simulink model "simscape_quadcopter_readtime_LQR_V1_2020a"  (R2022b)
settings: Solver=ode8  StartTime=0.0  StopTime=200  FixedStep=0.002  RelTol=1e-3
values from neighbouring files (symbols this model uses):
  C = [ 1  0  0  0  0  0 ... (first row only)    [LQR_QUADCOPTER_6STATE.m]    (also in LQR_QUADCOPTER_8STATE.m = [ 1     0     0     0     0     0     0     0)
  g = 9.81    [LQR_QUADCOPTER_6STATE.m]
  K_LQR_GOC = lqr(A,B,Q,R)    [LQR_QUADCOPTER_6STATE.m]
  m = 1.7    [LQR_QUADCOPTER_6STATE.m]
  pitch_init = 0    [LQR_QUADCOPTER_6STATE.m]    (also in LQR_QUADCOPTER_8STATE.m)
  roll_init = 0    [LQR_QUADCOPTER_6STATE.m]    (also in LQR_QUADCOPTER_8STATE.m)
  v_pitch_init = 0    [LQR_QUADCOPTER_6STATE.m]    (also in LQR_QUADCOPTER_8STATE.m)
  v_roll_init = 0    [LQR_QUADCOPTER_6STATE.m]    (also in LQR_QUADCOPTER_8STATE.m)
  v_x_init = 0    [LQR_QUADCOPTER_6STATE.m]    (also in LQR_QUADCOPTER_8STATE.m)
  v_y_init = 0    [LQR_QUADCOPTER_6STATE.m]    (also in LQR_QUADCOPTER_8STATE.m)
  v_yaw_init = 0    [LQR_QUADCOPTER_6STATE.m]    (also in LQR_QUADCOPTER_8STATE.m)
  v_z_init = 0    [LQR_QUADCOPTER_6STATE.m]    (also in LQR_QUADCOPTER_8STATE.m)
  x_init = 0    [LQR_QUADCOPTER_6STATE.m]    (also in LQR_QUADCOPTER_8STATE.m)
  y_init = 0    [LQR_QUADCOPTER_6STATE.m]    (also in LQR_QUADCOPTER_8STATE.m)
  yaw_init = 0    [LQR_QUADCOPTER_6STATE.m]    (also in LQR_QUADCOPTER_8STATE.m)
  z_init = 0    [LQR_QUADCOPTER_6STATE.m]    (also in LQR_QUADCOPTER_8STATE.m)
undefined symbols (not defined in the file or in its folder): drone_leg, X, Y, Z
libraries: sm_lib x55, nesl_utility x12, simulink x1
(part 1 of 2)
settings Model: Creator=tridu  LastModifiedBy=tridu
settings SolverCC: AlgebraicLoopSolver=TrustRegion
settings OptimizationCC: GainParamInheritBuiltInType=on

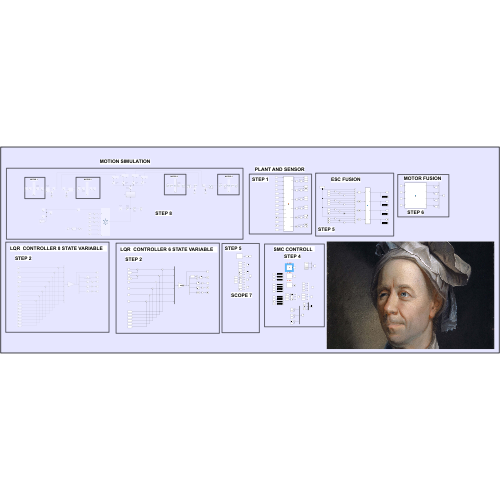
[thumbnail: Simulink's stored preview of the top-level diagram]
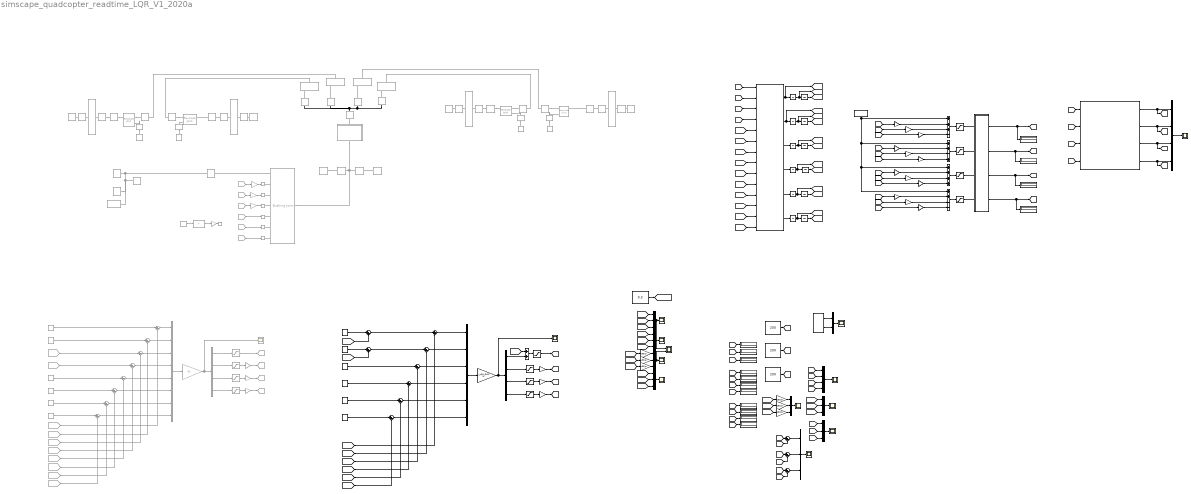
== system simscape_quadcopter_readtime_LQR_V1_2020a ==
  note: Z SP
  note: ARM 2
  note: ARM 2
  note: MOTOR 2
  note: MOTOR 3
  note: ARM 2
  note: MOTOR 1
  note: ARM 2
  note: ARM 2
  note: STEP 1
  note: STEP 5
  note: STEP 5
  note: MOTOR 4
  note: ARM 2
  note: SCOPE 7
  note: ARM 2
  note: ESC FUSION
  note: ARM 2
  note: STEP 8
  note: STEP 6
  note: PLANT AND SENSOR
  note: MOTION SIMULATION
  note: STEP 2
  note: LQR CONTROLLER 8 STATE VARIABLE
  note: ARM 2
  note: ARM 2
  note: MOTOR FUSION
  note: ARM 2
  note: STEP 2
  note: LQR CONTROLLER 6 STATE VARIABLE
  note: ARM 2
  note: SMC CONTROLL
  note: STEP 4
  note: X SP
  note: Y SP
  " Arm1" : sm_lib/Body Elements/File Solid  Commented=on  ExtGeomFileName=C:\Users\tridu\OneDrive\Máy tính\Code Matlad\quadcopter\CAD\Geometry\quadcopter_drone_arm.stp  UnitType=FromFile  ExtGeomFileUnits=m  StepReaderType=HEX  ExportConvexHullGeometry=off  InertiaType=Custom  Mass=0.0589152  MassUnits=kg  CenterOfMass=[-4.85019e-05, -0.00435236, -0.00536926]  CenterOfMassUnits=m  MomentsOfInertia=[0.000263222, 0.000260855, 1.23093e-05]  MomentsOfInertiaUnits=kg*m^2  ProductsOfInertia=[1.89459e-06, 5.49897e-08, 2.10429e-08]  ProductsOfInertiaUnits=kg*m^2  BasedOnType=Density  Density=1  DensityUnits=g/cm^3  DoExposeReferenceFrame=off  SerializedFrames=<Frames><Frame><Id>Frame1</Id><Value><Name>port</Name><Origin><Source>GeometricFeature</Source><FeatureName>planar surface 13</FeatureName></Origin><PrimaryAxis><DefinedDirection>-Z</DefinedDirection><Source>ReferenceFrame</Source><SourceDirection>+Z</SourceDirection><FeatureName></FeatureName></PrimaryAxis><SecondaryAxis><DefinedDirection>-X</DefinedDirection><Source>ReferenceFrame</Source><SourceDirection>+X</SourceDirection><FeatureName></FeatureName></SecondaryAxis></Value></Frame><Frame><Id>Frame2</Id><Value><Name>F2</Name><Origin><Source>GeometricFeature</Source><FeatureName>planar surface 4</FeatureName></Origin><PrimaryAxis><DefinedDirection>+Z</DefinedDirection><Source>ReferenceFrame</Source><SourceDirection>+Z</SourceDirection><FeatureName></FeatureName></PrimaryAxis><SecondaryAxis><DefinedDirection>+X</DefinedDirection><Source>ReferenceFrame</Source><SourceDirection>+X</SourceDirection><FeatureName></FeatureName></SecondaryAxis></Value></Frame><Frame><Id>Frame4</Id><Value><Name>Foot</Name><Origin><Source>GeometricFeature</Source><FeatureName>planar surface 62</FeatureName></Origin><PrimaryAxis><DefinedDirection>+Z</DefinedDirection><Source>ReferenceFrame</Source><SourceDirection>+Z</SourceDirection><FeatureName></FeatureName></PrimaryAxis><SecondaryAxis><DefinedDirection>+X</DefinedDirection><Source>ReferenceFrame</Source><SourceDirection>+X</SourceDirection><FeatureName></FeatureName></SecondaryAxis></Value></Frame></Frames>  GraphicType=FromGeometry  MarkerShape=Sphere  MarkerSize=10  GraphicVisPropType=SimpleVisualProperties  GraphicDiffuseColor=[1.0 0.0 0.2]  GraphicSpecularColor=[0.5 0.5 0.5 1.0]  GraphicAmbientColor=[0.15 0.15 0.15 1.0]  GraphicEmissiveColor=[0.0 0.0 0.0 1.0]  GraphicShininess=75  GraphicOpacity=1.0
  " Arm2" : sm_lib/Body Elements/File Solid  Commented=on  ExtGeomFileName=C:\Users\tridu\OneDrive\Máy tính\Code Matlad\quadcopter\CAD\Geometry\quadcopter_drone_arm.stp  UnitType=FromFile  ExtGeomFileUnits=m  StepReaderType=HEX  ExportConvexHullGeometry=off  InertiaType=Custom  Mass=0.0589152  MassUnits=kg  CenterOfMass=[-4.85019e-05, -0.00435236, -0.00536926]  CenterOfMassUnits=m  MomentsOfInertia=[0.000263222, 0.000260855, 1.23093e-05]  MomentsOfInertiaUnits=kg*m^2  ProductsOfInertia=[1.89459e-06, 5.49897e-08, 2.10429e-08]  ProductsOfInertiaUnits=kg*m^2  BasedOnType=Density  Density=1  DensityUnits=g/cm^3  DoExposeReferenceFrame=off  SerializedFrames=<Frames><Frame><Id>Frame1</Id><Value><Name>port</Name><Origin><Source>GeometricFeature</Source><FeatureName>planar surface 13</FeatureName></Origin><PrimaryAxis><DefinedDirection>-Z</DefinedDirection><Source>ReferenceFrame</Source><SourceDirection>+Z</SourceDirection><FeatureName></FeatureName></PrimaryAxis><SecondaryAxis><DefinedDirection>-X</DefinedDirection><Source>ReferenceFrame</Source><SourceDirection>+X</SourceDirection><FeatureName></FeatureName></SecondaryAxis></Value></Frame><Frame><Id>Frame2</Id><Value><Name>F2</Name><Origin><Source>GeometricFeature</Source><FeatureName>planar surface 4</FeatureName></Origin><PrimaryAxis><DefinedDirection>+Z</DefinedDirection><Source>ReferenceFrame</Source><SourceDirection>+Z</SourceDirection><FeatureName></FeatureName></PrimaryAxis><SecondaryAxis><DefinedDirection>+X</DefinedDirection><Source>ReferenceFrame</Source><SourceDirection>+X</SourceDirection><FeatureName></FeatureName></SecondaryAxis></Value></Frame><Frame><Id>Frame4</Id><Value><Name>Foot</Name><Origin><Source>GeometricFeature</Source><FeatureName>planar surface 62</FeatureName></Origin><PrimaryAxis><DefinedDirection>+Z</DefinedDirection><Source>ReferenceFrame</Source><SourceDirection>+Z</SourceDirection><FeatureName></FeatureName></PrimaryAxis><SecondaryAxis><DefinedDirection>+X</DefinedDirection><Source>ReferenceFrame</Source><SourceDirection>+X</SourceDirection><FeatureName></FeatureName></SecondaryAxis></Value></Frame></Frames>  GraphicType=FromGeometry  MarkerShape=Sphere  MarkerSize=10  GraphicVisPropType=SimpleVisualProperties  GraphicDiffuseColor=[1.0 0.0 0.2]  GraphicSpecularColor=[0.5 0.5 0.5 1.0]  GraphicAmbientColor=[0.15 0.15 0.15 1.0]  GraphicEmissiveColor=[0.0 0.0 0.0 1.0]  GraphicShininess=75  GraphicOpacity=1.0
  Add : Sum
  Add1 : Sum  Inputs=+++-
  Add3 : Sum  Inputs=++-+
  Add4 : Sum  Inputs=++++
  Add5 : Sum  Inputs=++--
  Arm1 : sm_lib/Body Elements/File Solid  Commented=on  ExtGeomFileName=C:\Users\tridu\OneDrive\Máy tính\Code Matlad\quadcopter\CAD\Geometry\quadcopter_drone_arm.stp  UnitType=FromFile  ExtGeomFileUnits=m  StepReaderType=HEX  ExportConvexHullGeometry=off  InertiaType=Custom  Mass=0.0589152  MassUnits=kg  CenterOfMass=[-4.85019e-05, -0.00435236, -0.00536926]  CenterOfMassUnits=m  MomentsOfInertia=[0.000263222, 0.000260855, 1.23093e-05]  MomentsOfInertiaUnits=kg*m^2  ProductsOfInertia=[1.89459e-06, 5.49897e-08, 2.10429e-08]  ProductsOfInertiaUnits=kg*m^2  BasedOnType=Density  Density=1  DensityUnits=g/cm^3  DoExposeReferenceFrame=off  SerializedFrames=<Frames><Frame><Id>Frame1</Id><Value><Name>port</Name><Origin><Source>GeometricFeature</Source><FeatureName>planar surface 13</FeatureName></Origin><PrimaryAxis><DefinedDirection>-Z</DefinedDirection><Source>ReferenceFrame</Source><SourceDirection>+Z</SourceDirection><FeatureName></FeatureName></PrimaryAxis><SecondaryAxis><DefinedDirection>-X</DefinedDirection><Source>ReferenceFrame</Source><SourceDirection>+X</SourceDirection><FeatureName></FeatureName></SecondaryAxis></Value></Frame><Frame><Id>Frame2</Id><Value><Name>F2</Name><Origin><Source>GeometricFeature</Source><FeatureName>planar surface 4</FeatureName></Origin><PrimaryAxis><DefinedDirection>+Z</DefinedDirection><Source>ReferenceFrame</Source><SourceDirection>+Z</SourceDirection><FeatureName></FeatureName></PrimaryAxis><SecondaryAxis><DefinedDirection>+X</DefinedDirection><Source>ReferenceFrame</Source><SourceDirection>+X</SourceDirection><FeatureName></FeatureName></SecondaryAxis></Value></Frame><Frame><Id>Frame3</Id><Value><Name>Foot</Name><Origin><Source>GeometricFeature</Source><FeatureName>planar surface 62</FeatureName></Origin><PrimaryAxis><DefinedDirection>+Z</DefinedDirection><Source>ReferenceFrame</Source><SourceDirection>+Z</SourceDirection><FeatureName></FeatureName></PrimaryAxis><SecondaryAxis><DefinedDirection>+X</DefinedDirection><Source>ReferenceFrame</Source><SourceDirection>+X</SourceDirection><FeatureName></FeatureName></SecondaryAxis></Value></Frame></Frames>  GraphicType=FromGeometry  MarkerShape=Sphere  MarkerSize=10  GraphicVisPropType=SimpleVisualProperties  GraphicDiffuseColor=[1.0 1.0 1.0]  GraphicSpecularColor=[0.5 0.5 0.5 1.0]  GraphicAmbientColor=[0.15 0.15 0.15 1.0]  GraphicEmissiveColor=[0.0 0.0 0.0 1.0]  GraphicShininess=75  GraphicOpacity=1.0
  Arm2 : sm_lib/Body Elements/File Solid  Commented=on  ExtGeomFileName=C:\Users\tridu\OneDrive\Máy tính\Code Matlad\quadcopter\CAD\Geometry\quadcopter_drone_arm.stp  UnitType=FromFile  ExtGeomFileUnits=m  StepReaderType=HEX  ExportConvexHullGeometry=off  InertiaType=Custom  Mass=0.0589152  MassUnits=kg  CenterOfMass=[-4.85019e-05, -0.00435236, -0.00536926]  CenterOfMassUnits=m  MomentsOfInertia=[0.000263222, 0.000260855, 1.23093e-05]  MomentsOfInertiaUnits=kg*m^2  ProductsOfInertia=[1.89459e-06, 5.49897e-08, 2.10429e-08]  ProductsOfInertiaUnits=kg*m^2  BasedOnType=Density  Density=1  DensityUnits=g/cm^3  DoExposeReferenceFrame=off  SerializedFrames=<Frames><Frame><Id>Frame1</Id><Value><Name>port</Name><Origin><Source>GeometricFeature</Source><FeatureName>planar surface 13</FeatureName></Origin><PrimaryAxis><DefinedDirection>-Z</DefinedDirection><Source>ReferenceFrame</Source><SourceDirection>+Z</SourceDirection><FeatureName></FeatureName></PrimaryAxis><SecondaryAxis><DefinedDirection>-X</DefinedDirection><Source>ReferenceFrame</Source><SourceDirection>+X</SourceDirection><FeatureName></FeatureName></SecondaryAxis></Value></Frame><Frame><Id>Frame2</Id><Value><Name>F2</Name><Origin><Source>GeometricFeature</Source><FeatureName>planar surface 4</FeatureName></Origin><PrimaryAxis><DefinedDirection>+Z</DefinedDirection><Source>ReferenceFrame</Source><SourceDirection>+Z</SourceDirection><FeatureName></FeatureName></PrimaryAxis><SecondaryAxis><DefinedDirection>+X</DefinedDirection><Source>ReferenceFrame</Source><SourceDirection>+X</SourceDirection><FeatureName></FeatureName></SecondaryAxis></Value></Frame><Frame><Id>Frame3</Id><Value><Name>Foot</Name><Origin><Source>GeometricFeature</Source><FeatureName>planar surface 62</FeatureName></Origin><PrimaryAxis><DefinedDirection>+Z</DefinedDirection><Source>ReferenceFrame</Source><SourceDirection>+Z</SourceDirection><FeatureName></FeatureName></PrimaryAxis><SecondaryAxis><DefinedDirection>+X</DefinedDirection><Source>ReferenceFrame</Source><SourceDirection>+X</SourceDirection><FeatureName></FeatureName></SecondaryAxis></Value></Frame></Frames>  GraphicType=FromGeometry  MarkerShape=Sphere  MarkerSize=10  GraphicVisPropType=SimpleVisualProperties  GraphicDiffuseColor=[1.0 1.0 1.0]  GraphicSpecularColor=[0.5 0.5 0.5 1.0]  GraphicAmbientColor=[0.15 0.15 0.15 1.0]  GraphicEmissiveColor=[0.0 0.0 0.0 1.0]  GraphicShininess=75  GraphicOpacity=1.0
  Body : Subsystem  Commented=on
  Bushing Joint : sm_lib/Joints/Bushing Joint  Commented=on  JointMode=Normal  SenseConstraintForce=off  SenseConstraintForceX=off  SenseConstraintForceY=off  SenseConstraintForceZ=off  SenseConstraintTorque=off  SenseConstraintTorqueX=off  SenseConstraintTorqueY=off  SenseConstraintTorqueZ=off  SenseTotalForce=off  SenseTotalForceX=off  SenseTotalForceY=off  SenseTotalForceZ=off  SenseTotalTorque=off  SenseTotalTorqueX=off  SenseTotalTorqueY=off  SenseTotalTorqueZ=off  CompositeWrenchDir=FollowerOnBase  CompositeWrenchFrame=BaseFrame  PxEquilibriumPosition=0  PxEquilibriumPositionUnits=m  PxSpringStiffness=0  PxSpringStiffnessUnits=N/m  PxDampingCoefficient=0  PxDampingCoefficientUnits=N/(m/s)  PxTorqueActuationMode=ComputedTorque  PxMotionActuationMode=InputMotion  PxSensePosition=off  PxSenseVelocity=off  PxSenseAcceleration=off  PxSenseTorqueForce=off  PxSenseLowerLimitTorqueForce=off  PxSenseUpperLimitTorqueForce=off  PxLowerLimitSpecify=off  PxLowerLimitBound=-1  PxLowerLimitBoundUnits=m  PxLowerLimitStiffness=1e6  PxLowerLimitStiffnessUnits=N/m  PxLowerLimitDamping=1e3  PxLowerLimitDampingUnits=N/(m/s)  PxLowerLimitTransitionRegionWidth=1e-4  PxLowerLimitTransitionRegionWidthUnits=m  PxUpperLimitSpecify=off  PxUpperLimitBound=1  PxUpperLimitBoundUnits=m  PxUpperLimitStiffness=1e6  PxUpperLimitStiffnessUnits=N/m  PxUpperLimitDamping=1e3  PxUpperLimitDampingUnits=N/(m/s)  PxUpperLimitTransitionRegionWidth=1e-4  PxUpperLimitTransitionRegionWidthUnits=m  PxPositionTargetSpecify=off  PxPositionTargetPriority=High  PxPositionTargetValue=0  PxPositionTargetValueUnits=m  PxVelocityTargetSpecify=off  PxVelocityTargetPriority=High  PxVelocityTargetValue=0  PxVelocityTargetValueUnits=m/s  PyEquilibriumPosition=0  PyEquilibriumPositionUnits=m  PySpringStiffness=0  PySpringStiffnessUnits=N/m  PyDampingCoefficient=0  PyDampingCoefficientUnits=N/(m/s)  PyTorqueActuationMode=ComputedTorque  PyMotionActuationMode=InputMotion  PySensePosition=off  PySenseVelocity=off  PySenseAcceleration=off  PySenseTorqueForce=off  PySenseLowerLimitTorqueForce=off  PySenseUpperLimitTorqueForce=off  PyLowerLimitSpecify=off  PyLowerLimitBound=-1  PyLowerLimitBoundUnits=m  PyLowerLimitStiffness=1e6  PyLowerLimitStiffnessUnits=N/m  PyLowerLimitDamping=1e3  PyLowerLimitDampingUnits=N/(m/s)  PyLowerLimitTransitionRegionWidth=1e-4  PyLowerLimitTransitionRegionWidthUnits=m  PyUpperLimitSpecify=off  PyUpperLimitBound=1  PyUpperLimitBoundUnits=m  PyUpperLimitStiffness=1e6  PyUpperLimitStiffnessUnits=N/m  PyUpperLimitDamping=1e3  PyUpperLimitDampingUnits=N/(m/s)  PyUpperLimitTransitionRegionWidth=1e-4  PyUpperLimitTransitionRegionWidthUnits=m  PyPositionTargetSpecify=off  PyPositionTargetPriority=High  PyPositionTargetValue=0  PyPositionTargetValueUnits=m  PyVelocityTargetSpecify=off  PyVelocityTargetPriority=High  PyVelocityTargetValue=0  PyVelocityTargetValueUnits=m/s  PzEquilibriumPosition=0  PzEquilibriumPositionUnits=m  PzSpringStiffness=0  PzSpringStiffnessUnits=N/m  PzDampingCoefficient=0  PzDampingCoefficientUnits=N/(m/s)  PzTorqueActuationMode=ComputedTorque  PzMotionActuationMode=InputMotion  PzSensePosition=off  PzSenseVelocity=off  PzSenseAcceleration=off  PzSenseTorqueForce=off  PzSenseLowerLimitTorqueForce=off  PzSenseUpperLimitTorqueForce=off  PzLowerLimitSpecify=off  PzLowerLimitBound=-1  PzLowerLimitBoundUnits=m  PzLowerLimitStiffness=1e6  PzLowerLimitStiffnessUnits=N/m  PzLowerLimitDamping=1e3  PzLowerLimitDampingUnits=N/(m/s)  PzLowerLimitTransitionRegionWidth=1e-4  PzLowerLimitTransitionRegionWidthUnits=m  PzUpperLimitSpecify=off  PzUpperLimitBound=1  PzUpperLimitBoundUnits=m  PzUpperLimitStiffness=1e6  PzUpperLimitStiffnessUnits=N/m  PzUpperLimitDamping=1e3  PzUpperLimitDampingUnits=N/(m/s)  PzUpperLimitTransitionRegionWidth=1e-4  PzUpperLimitTransitionRegionWidthUnits=m  PzPositionTargetSpecify=off  PzPositionTargetPriority=High  PzPositionTargetValue=0  PzPositionTargetValueUnits=m  PzVelocityTargetSpecify=off  PzVelocityTargetPriority=High  PzVelocityTargetValue=0  PzVelocityTargetValueUnits=m/s  RxEquilibriumPosition=0  RxEquilibriumPositionUnits=deg  RxSpringStiffness=0  RxSpringStiffnessUnits=N*m/deg  RxDampingCoefficient=0  RxDampingCoefficientUnits=N*m/(deg/s)  RxTorqueActuationMode=ComputedTorque  RxMotionActuationMode=InputMotion  RxSensePosition=off  RxSenseVelocity=off  RxSenseAcceleration=off  RxSenseTorqueForce=off  RxSenseLowerLimitTorqueForce=off  RxSenseUpperLimitTorqueForce=off  RxLowerLimitSpecify=off  RxLowerLimitBound=-90  RxLowerLimitBoundUnits=deg  RxLowerLimitStiffness=1e4  RxLowerLimitStiffnessUnits=N*m/deg  RxLowerLimitDamping=10  RxLowerLimitDampingUnits=N*m/(deg/s)  RxLowerLimitTransitionRegionWidth=0.1  RxLowerLimitTransitionRegionWidthUnits=deg  RxUpperLimitSpecify=off  RxUpperLimitBound=90  RxUpperLimitBoundUnits=deg  RxUpperLimitStiffness=1e4  RxUpperLimitStiffnessUnits=N*m/deg  RxUpperLimitDamping=10  RxUpperLimitDampingUnits=N*m/(deg/s)  RxUpperLimitTransitionRegionWidth=0.1  RxUpperLimitTransitionRegionWidthUnits=deg  RxPositionTargetSpecify=off  RxPositionTargetPriority=High  RxPositionTargetValue=0  RxPositionTargetValueUnits=deg  RxVelocityTargetSpecify=off  RxVelocityTargetPriority=High  RxVelocityTargetValue=0  RxVelocityTargetValueUnits=deg/s  RyEquilibriumPosition=0  RyEquilibriumPositionUnits=deg  RySpringStiffness=0  RySpringStiffnessUnits=N*m/deg  RyDampingCoefficient=0  RyDampingCoefficientUnits=N*m/(deg/s)  RyTorqueActuationMode=ComputedTorque  RyMotionActuationMode=InputMotion  RySensePosition=off  RySenseVelocity=off  RySenseAcceleration=off  RySenseTorqueForce=off  RySenseLowerLimitTorqueForce=off  RySenseUpperLimitTorqueForce=off  RyLowerLimitSpecify=off  RyLowerLimitBound=-90  RyLowerLimitBoundUnits=deg  RyLowerLimitStiffness=1e4  RyLowerLimitStiffnessUnits=N*m/deg  RyLowerLimitDamping=10  RyLowerLimitDampingUnits=N*m/(deg/s)  RyLowerLimitTransitionRegionWidth=0.1  RyLowerLimitTransitionRegionWidthUnits=deg  RyUpperLimitSpecify=off  RyUpperLimitBound=90  RyUpperLimitBoundUnits=deg  RyUpperLimitStiffness=1e4  RyUpperLimitStiffnessUnits=N*m/deg  RyUpperLimitDamping=10  RyUpperLimitDampingUnits=N*m/(deg/s)  RyUpperLimitTransitionRegionWidth=0.1  RyUpperLimitTransitionRegionWidthUnits=deg  RyPositionTargetSpecify=off  RyPositionTargetPriority=High  RyPositionTargetValue=0  RyPositionTargetValueUnits=deg  RyVelocityTargetSpecify=off  RyVelocityTargetPriority=High  RyVelocityTargetValue=0  RyVelocityTargetValueUnits=deg/s  RzEquilibriumPosition=0  RzEquilibriumPositionUnits=deg  RzSpringStiffness=0  RzSpringStiffnessUnits=N*m/deg  RzDampingCoefficient=0  RzDampingCoefficientUnits=N*m/(deg/s)  RzTorqueActuationMode=ComputedTorque  RzMotionActuationMode=InputMotion  RzSensePosition=off  RzSenseVelocity=off  RzSenseAcceleration=off  RzSenseTorqueForce=off  RzSenseLowerLimitTorqueForce=off  RzSenseUpperLimitTorqueForce=off  RzLowerLimitSpecify=off  RzLowerLimitBound=-90  RzLowerLimitBoundUnits=deg  RzLowerLimitStiffness=1e4  RzLowerLimitStiffnessUnits=N*m/deg  RzLowerLimitDamping=10  RzLowerLimitDampingUnits=N*m/(deg/s)  RzLowerLimitTransitionRegionWidth=0.1  RzLowerLimitTransitionRegionWidthUnits=deg  RzUpperLimitSpecify=off  RzUpperLimitBound=90  RzUpperLimitBoundUnits=deg  RzUpperLimitStiffness=1e4  RzUpperLimitStiffnessUnits=N*m/deg  RzUpperLimitDamping=10  RzUpperLimitDampingUnits=N*m/(deg/s)  RzUpperLimitTransitionRegionWidth=0.1  RzUpperLimitTransitionRegionWidthUnits=deg  RzPositionTargetSpecify=off  RzPositionTargetPriority=High  RzPositionTargetValue=0  RzPositionTargetValueUnits=deg  RzVelocityTargetSpecify=off  RzVelocityTargetPriority=High  RzVelocityTargetValue=0  RzVelocityTargetValueUnits=deg/s
  Cap{1..4} (4 alike) : sm_lib/Body Elements/File Solid  Commented=on  ExtGeomFileName=C:\Users\tridu\OneDrive\Máy tính\Code Matlad\quadcopter\CAD\Geometry\quadcopter_drone_motor_cap.stp  UnitType=FromFile  ExtGeomFileUnits=m  StepReaderType=HEX  ExportConvexHullGeometry=off  InertiaType=Custom  Mass=0.000930841  MassUnits=kg  CenterOfMass=[0 0.00200877 0]  CenterOfMassUnits=m  MomentsOfInertia=[1.32154e-08, 2.22535e-08, 1.32154e-08]  MomentsOfInertiaUnits=kg*m^2  ProductsOfInertia=[0 0 0]  ProductsOfInertiaUnits=kg*m^2  BasedOnType=Density  Density=1  DensityUnits=g/cm^3  DoExposeReferenceFrame=on  SerializedFrames=<Frames/>  GraphicType=FromGeometry  MarkerShape=Sphere  MarkerSize=10  GraphicVisPropType=AdvancedVisualProperties  GraphicDiffuseColor=[0.05 0.05 0.05]  GraphicSpecularColor=[0.5 0.5 0.5 1.0]  GraphicAmbientColor=[0.15 0.15 0.15 1.0]  GraphicEmissiveColor=[0.0 0.0 0.0 1.0]  GraphicShininess=40  GraphicOpacity=1.0
  Constant : Constant  Value=1.7*9.81/4
  Constant1 : Constant  Commented=on  Value=-1
  Constant13 : Constant  Commented=on  Value=100
  Constant{4,14..17} (5 alike) : Constant  Commented=on  Value=0
  Constant{2..3,23,25..27} (6 alike) : Constant  Value=0
  Constant28 : Constant  Commented=on
  Constant29 : Constant  Value=200
  Constant31 : Constant  Value=200
  Constant36 : Constant  Value=200
  Constant37 : Constant  Commented=on
  Constant38 : Constant  Commented=on
  Constant7 : Constant  Commented=on  Value=-1
  Demux1 : Demux  Commented=on
  Demux2 : Demux
  Display{,1..10,14..17} (15 alike) : Display
  From18 : From  Commented=on  GotoTag=z  TagVisibility=global
  From19 : From  Commented=on  GotoTag=roll  TagVisibility=global
  From20 : From  Commented=on  GotoTag=pitch  TagVisibility=global
  From21 : From  Commented=on  GotoTag=yaw  TagVisibility=global
  From22 : From  Commented=on  GotoTag=roll  TagVisibility=global
  From23 : From  Commented=on  GotoTag=yawdot  TagVisibility=global
  From24 : From  Commented=on  GotoTag=x  TagVisibility=global
  From25 : From  Commented=on  GotoTag=y  TagVisibility=global
  From26 : From  Commented=on  GotoTag=pitchdot  TagVisibility=global
  From27 : From  Commented=on  GotoTag=rolldot  TagVisibility=global
  From28 : From  Commented=on  GotoTag=yaw  TagVisibility=global
  From29 : From  Commented=on  GotoTag=pitch  TagVisibility=global
  From57 : From  Commented=on  GotoTag=zdot  TagVisibility=global
  From60 : From  Commented=on  GotoTag=z  TagVisibility=global
  From71 : From  Commented=on  GotoTag=roll_SP  TagVisibility=global
  From72 : From  Commented=on  GotoTag=pitch_SP  TagVisibility=global
  Gain1 : Gain  Commented=on  Gain=1/110
  Gain{8..12,14,16,18} (8 alike) : Gain  Gain=1/4
  Gain{13,15,17,19} (4 alike) : Gain  Gain=1/2
  Gain2 : Gain  Commented=on  Gain=1/100
  Gain20 : Gain  Gain=0.3
  Gain21 : Gain  Commented=on  Gain=|  Multiplication=Matrix(K*u)
      | [3.1623    7.7943   -0.0000   -0.0000    0.0000   -0.0000   -0.0000    0.0000;
      |       -0.0000   -0.0000    3.1623   -0.0000    0.0000    1.0033   -0.0000    0.0000;
      |        0.0000   -0.0000   -0.0000    3.1623   -0.0000   -0.0000    1.0033   -0.0000;
      |        0.0000   -0.0000   -0.0000    0.0000    3.1623   -0.0000    0.0000    1.0043]
  Gain22 : Gain  Commented=on  Gain=0.3
  Gain23 : Gain  Commented=on  Gain=0.3
  Gain24 : Gain  Gain=0.3
  Gain25 : Gain  Commented=on  Gain=0.1
  Gain26 : Gain  Gain=0.1
  Gain27 : Gain  Commented=on  Gain=1/100
  Gain{4..6,28..30} (6 alike) : Gain  Gain=180/pi
  Gain3 : Gain  Commented=on  Gain=1/100
  Gain7 : Gain  Gain=K_LQR_GOC  Multiplication=Matrix(K*u)
  Giới hạn công suất U1 : Saturate  Commented=on  UpperLimit=29.3230*0.3  LowerLimit=-1.7*9.81
  Giới hạn công suất U2 : Saturate  UpperLimit=29.3230  LowerLimit=-1.7*9.81
  Goto21 : Goto  Commented=on  GotoTag=U1  TagVisibility=global
  Goto22 : Goto  Commented=on  GotoTag=U2  TagVisibility=global
  Goto23 : Goto  Commented=on  GotoTag=U3  TagVisibility=global
  Goto29 : Goto  Commented=on  GotoTag=U4  TagVisibility=global
  HS_MSKK : Constant  Value=0.3
  Housing{1..4} (4 alike) : sm_lib/Body Elements/File Solid  Commented=on  ExtGeomFileName=C:\Users\tridu\OneDrive\Máy tính\Code Matlad\quadcopter\CAD\Geometry\quadcopter_drone_motor.stp  UnitType=FromFile  ExtGeomFileUnits=m  StepReaderType=HEX  ExportConvexHullGeometry=off  InertiaType=Custom  Mass=51  MassUnits=g  CenterOfMass=[0, 0, -0.0088876]  CenterOfMassUnits=m  MomentsOfInertia=[7.0438e-06, 7.04379e-06, 6.06908e-06]  MomentsOfInertiaUnits=kg*m^2  ProductsOfInertia=[0 0 0]  ProductsOfInertiaUnits=kg*m^2  BasedOnType=Mass  Density=1000  DensityUnits=kg/m^3  DoExposeReferenceFrame=on  SerializedFrames=<Frames><Frame><Id>Frame1</Id><Value><Name>F1</Name><Origin><Source>CenterOfMassFrame</Source><FeatureName></FeatureName></Origin><PrimaryAxis><DefinedDirection>-Z</DefinedDirection><Source>ReferenceFrame</Source><SourceDirection>+Z</SourceDirection><FeatureName></FeatureName></PrimaryAxis><SecondaryAxis><DefinedDirection>+X</DefinedDirection><Source>ReferenceFrame</Source><SourceDirection>+X</SourceDirection><FeatureName></FeatureName></SecondaryAxis></Value></Frame></Frames>  GraphicType=FromGeometry  MarkerShape=Sphere  MarkerSize=10  GraphicVisPropType=SimpleVisualProperties  GraphicDiffuseColor=[0.6 0.0 0.2]  GraphicSpecularColor=[0.5 0.5 0.5 1.0]  GraphicAmbientColor=[0.15 0.15 0.15 1.0]  GraphicEmissiveColor=[0.0 0.0 0.0 1.0]  GraphicShininess=75  GraphicOpacity=1.0
  Integrator : Integrator  InitialCondition=v_x_init
  Integrator1 : Integrator  InitialCondition=x_init
  Integrator10 : Integrator  InitialCondition=v_yaw_init
  Integrator11 : Integrator  InitialCondition=yaw_init
  Integrator2 : Integrator  InitialCondition=v_y_init
  Integrator3 : Integrator  InitialCondition=y_init
  Integrator4 : Integrator  InitialCondition=z_init
  Integrator5 : Integrator  InitialCondition=v_z_init
  Integrator6 : Integrator  InitialCondition=v_roll_init
  Integrator7 : Integrator  InitialCondition=roll_init
  Integrator8 : Integrator  InitialCondition=v_pitch_init
  Integrator9 : Integrator  InitialCondition=pitch_init
  MATLAB Function : MATLAB Function  TreatAsAtomicUnit=on
  MATLAB Function1 : MATLAB Function  TreatAsAtomicUnit=on
  MATLAB Function2 : MATLAB Function  TreatAsAtomicUnit=on
  MechanismConfiguration : sm_lib/Utilities/Mechanism Configuration  Commented=on  UniformGravity=Constant  GravityVector=[0 -9.81 0]  GravityUnits=m/s^2  LinearizationDelta=0.002  JointModeTransitionNonlinearIterations=2
  Mux{,1..3,13..16} (8 alike) : Mux  Inputs=3
  Mux10 : Mux  Inputs=6
  Mux11 : Mux
  Mux12 : Mux  Inputs=2
  Mux4 : Mux
  Mux5 : Mux  Commented=on  Inputs=8
  Propeller1 : sm_lib/Body Elements/File Solid  Commented=on  ExtGeomFileName=C:\Users\tridu\OneDrive\Máy tính\Code Matlad\quadcopter\CAD\Geometry\quadcopter_drone_propeller_1_4.stp  UnitType=FromFile  ExtGeomFileUnits=m  StepReaderType=HEX  ExportConvexHullGeometry=off  InertiaType=Custom  Mass=0.0249468  MassUnits=kg  CenterOfMass="[0  0.00566766 0]"  CenterOfMassUnits=m  MomentsOfInertia=[0.000160013, 0.000160582, 8.20018e-07]  MomentsOfInertiaUnits=kg*m^2  ProductsOfInertia=[0 0 0]  ProductsOfInertiaUnits=kg*m^2  BasedOnType=Density  Density=1  DensityUnits=g/cm^3  DoExposeReferenceFrame=on  SerializedFrames=<Frames><Frame><Id>Frame1</Id><Value><Name>R2</Name><Origin><Source>ReferenceFrame</Source><FeatureName></FeatureName></Origin><PrimaryAxis><DefinedDirection>+Z</DefinedDirection><Source>ReferenceFrame</Source><SourceDirection>+Z</SourceDirection><FeatureName></FeatureName></PrimaryAxis><SecondaryAxis><DefinedDirection>+X</DefinedDirection><Source>ReferenceFrame</Source><SourceDirection>+X</SourceDirection><FeatureName></FeatureName></SecondaryAxis></Value></Frame></Frames>  GraphicType=FromGeometry  MarkerShape=Sphere  MarkerSize=10  GraphicVisPropType=AdvancedVisualProperties  GraphicDiffuseColor=[0.05 0.05 0.05]  GraphicSpecularColor=[0.5 0.5 0.5 1.0]  GraphicAmbientColor=[0.15 0.15 0.15 1.0]  GraphicEmissiveColor=[0.0 0.0 0.0 1.0]  GraphicShininess=40  GraphicOpacity=1.0
  Propeller2 : sm_lib/Body Elements/File Solid  Commented=on  ExtGeomFileName=C:\Users\tridu\OneDrive\Máy tính\Code Matlad\quadcopter\CAD\Geometry\quadcopter_drone_propeller_2_3.stp  UnitType=FromFile  ExtGeomFileUnits=m  StepReaderType=HEX  ExportConvexHullGeometry=off  InertiaType=Custom  Mass=0.0249468  MassUnits=kg  CenterOfMass="[0  0.00566766 0]"  CenterOfMassUnits=m  MomentsOfInertia=[0.000160013, 0.000160582, 8.20018e-07]  MomentsOfInertiaUnits=kg*m^2  ProductsOfInertia=[0 0 0]  ProductsOfInertiaUnits=kg*m^2  BasedOnType=Density  Density=1  DensityUnits=g/cm^3  DoExposeReferenceFrame=on  SerializedFrames=<Frames><Frame><Id>Frame1</Id><Value><Name>R2</Name><Origin><Source>ReferenceFrame</Source><FeatureName></FeatureName></Origin><PrimaryAxis><DefinedDirection>+Z</DefinedDirection><Source>ReferenceFrame</Source><SourceDirection>+Z</SourceDirection><FeatureName></FeatureName></PrimaryAxis><SecondaryAxis><DefinedDirection>+X</DefinedDirection><Source>ReferenceFrame</Source><SourceDirection>+X</SourceDirection><FeatureName></FeatureName></SecondaryAxis></Value></Frame></Frames>  GraphicType=FromGeometry  MarkerShape=Sphere  MarkerSize=10  GraphicVisPropType=AdvancedVisualProperties  GraphicDiffuseColor=[0.05 0.05 0.05]  GraphicSpecularColor=[0.5 0.5 0.5 1.0]  GraphicAmbientColor=[0.15 0.15 0.15 1.0]  GraphicEmissiveColor=[0.0 0.0 0.0 1.0]  GraphicShininess=40  GraphicOpacity=1.0
  Propeller3 : sm_lib/Body Elements/File Solid  Commented=on  ExtGeomFileName=C:\Users\tridu\OneDrive\Máy tính\Code Matlad\quadcopter\CAD\Geometry\quadcopter_drone_propeller_2_3.stp  UnitType=FromFile  ExtGeomFileUnits=m  StepReaderType=HEX  ExportConvexHullGeometry=off  InertiaType=Custom  Mass=0.0249468  MassUnits=kg  CenterOfMass="[0  0.00566766 0]"  CenterOfMassUnits=m  MomentsOfInertia=[0.000160013, 0.000160582, 8.20018e-07]  MomentsOfInertiaUnits=kg*m^2  ProductsOfInertia=[0 0 0]  ProductsOfInertiaUnits=kg*m^2  BasedOnType=Density  Density=1  DensityUnits=g/cm^3  DoExposeReferenceFrame=on  SerializedFrames=<Frames><Frame><Id>Frame1</Id><Value><Name>R2</Name><Origin><Source>ReferenceFrame</Source><FeatureName></FeatureName></Origin><PrimaryAxis><DefinedDirection>+Z</DefinedDirection><Source>ReferenceFrame</Source><SourceDirection>+Z</SourceDirection><FeatureName></FeatureName></PrimaryAxis><SecondaryAxis><DefinedDirection>+X</DefinedDirection><Source>ReferenceFrame</Source><SourceDirection>+X</SourceDirection><FeatureName></FeatureName></SecondaryAxis></Value></Frame></Frames>  GraphicType=FromGeometry  MarkerShape=Sphere  MarkerSize=10  GraphicVisPropType=AdvancedVisualProperties  GraphicDiffuseColor=[0.05 0.05 0.05]  GraphicSpecularColor=[0.5 0.5 0.5 1.0]  GraphicAmbientColor=[0.15 0.15 0.15 1.0]  GraphicEmissiveColor=[0.0 0.0 0.0 1.0]  GraphicShininess=40  GraphicOpacity=1.0
  Propeller4 : sm_lib/Body Elements/File Solid  Commented=on  ExtGeomFileName=C:\Users\tridu\OneDrive\Máy tính\Code Matlad\quadcopter\CAD\Geometry\quadcopter_drone_propeller_1_4.stp  UnitType=FromFile  ExtGeomFileUnits=m  StepReaderType=HEX  ExportConvexHullGeometry=off  InertiaType=Custom  Mass=0.0249468  MassUnits=kg  CenterOfMass="[0  0.00566766 0]"  CenterOfMassUnits=m  MomentsOfInertia=[0.000160013, 0.000160582, 8.20018e-07]  MomentsOfInertiaUnits=kg*m^2  ProductsOfInertia=[0 0 0]  ProductsOfInertiaUnits=kg*m^2  BasedOnType=Density  Density=1  DensityUnits=g/cm^3  DoExposeReferenceFrame=on  SerializedFrames=<Frames><Frame><Id>Frame1</Id><Value><Name>R2</Name><Origin><Source>ReferenceFrame</Source><FeatureName></FeatureName></Origin><PrimaryAxis><DefinedDirection>+Z</DefinedDirection><Source>ReferenceFrame</Source><SourceDirection>+Z</SourceDirection><FeatureName></FeatureName></PrimaryAxis><SecondaryAxis><DefinedDirection>+X</DefinedDirection><Source>ReferenceFrame</Source><SourceDirection>+X</SourceDirection><FeatureName></FeatureName></SecondaryAxis></Value></Frame></Frames>  GraphicType=FromGeometry  MarkerShape=Sphere  MarkerSize=10  GraphicVisPropType=AdvancedVisualProperties  GraphicDiffuseColor=[0.05 0.05 0.05]  GraphicSpecularColor=[0.5 0.5 0.5 1.0]  GraphicAmbientColor=[0.15 0.15 0.15 1.0]  GraphicEmissiveColor=[0.0 0.0 0.0 1.0]  GraphicShininess=40  GraphicOpacity=1.0
  Revolute Joint3 : sm_lib/Joints/Revolute Joint  Commented=on  JointMode=Normal  SenseConstraintForce=off  SenseConstraintForceX=off  SenseConstraintForceY=off  SenseConstraintForceZ=off  SenseConstraintTorque=off  SenseConstraintTorqueX=off  SenseConstraintTorqueY=off  SenseConstraintTorqueZ=off  SenseTotalForce=off  SenseTotalForceX=off  SenseTotalForceY=off  SenseTotalForceZ=off  SenseTotalTorque=off  SenseTotalTorqueX=off  SenseTotalTorqueY=off  SenseTotalTorqueZ=off  CompositeWrenchDir=FollowerOnBase  CompositeWrenchFrame=BaseFrame  EquilibriumPosition=0  EquilibriumPositionUnits=deg  SpringStiffness=0  SpringStiffnessUnits=N*m/rad  DampingCoefficient=1e-5  DampingCoefficientUnits=N*m/(rad/s)  TorqueActuationMode=InputTorque  MotionActuationMode=ComputedMotion  SensePosition=off  SenseVelocity=on  SenseAcceleration=off  SenseTorqueForce=off  SenseLowerLimitTorqueForce=off  SenseUpperLimitTorqueForce=off  LowerLimitSpecify=off  LowerLimitBound=-90  LowerLimitBoundUnits=deg  LowerLimitStiffness=1e4  LowerLimitStiffnessUnits=N*m/deg  LowerLimitDamping=10  LowerLimitDampingUnits=N*m/(deg/s)  LowerLimitTransitionRegionWidth=0.1  LowerLimitTransitionRegionWidthUnits=deg  UpperLimitSpecify=off  UpperLimitBound=90  UpperLimitBoundUnits=deg  UpperLimitStiffness=1e4  UpperLimitStiffnessUnits=N*m/deg  UpperLimitDamping=10  UpperLimitDampingUnits=N*m/(deg/s)  UpperLimitTransitionRegionWidth=0.1  UpperLimitTransitionRegionWidthUnits=deg  PositionTargetSpecify=off  PositionTargetPriority=High  PositionTargetValue=0  PositionTargetValueUnits=deg  VelocityTargetSpecify=off  VelocityTargetPriority=High  VelocityTargetValue=0  VelocityTargetValueUnits=deg/s
  Revolute Joint : sm_lib/Joints/Revolute Joint  Commented=on  JointMode=Normal  SenseConstraintForce=off  SenseConstraintForceX=off  SenseConstraintForceY=off  SenseConstraintForceZ=off  SenseConstraintTorque=off  SenseConstraintTorqueX=off  SenseConstraintTorqueY=off  SenseConstraintTorqueZ=off  SenseTotalForce=off  SenseTotalForceX=off  SenseTotalForceY=off  SenseTotalForceZ=off  SenseTotalTorque=off  SenseTotalTorqueX=off  SenseTotalTorqueY=off  SenseTotalTorqueZ=off  CompositeWrenchDir=FollowerOnBase  CompositeWrenchFrame=BaseFrame  EquilibriumPosition=0  EquilibriumPositionUnits=deg  SpringStiffness=0  SpringStiffnessUnits=N*m/deg  DampingCoefficient=0  DampingCoefficientUnits=N*m/(deg/s)  TorqueActuationMode=InputTorque  MotionActuationMode=ComputedMotion  SensePosition=off  SenseVelocity=on  SenseAcceleration=off  SenseTorqueForce=off  SenseLowerLimitTorqueForce=off  SenseUpperLimitTorqueForce=off  LowerLimitSpecify=off  LowerLimitBound=-90  LowerLimitBoundUnits=deg  LowerLimitStiffness=1e4  LowerLimitStiffnessUnits=N*m/deg  LowerLimitDamping=10  LowerLimitDampingUnits=N*m/(deg/s)  LowerLimitTransitionRegionWidth=0.1  LowerLimitTransitionRegionWidthUnits=deg  UpperLimitSpecify=off  UpperLimitBound=90  UpperLimitBoundUnits=deg  UpperLimitStiffness=1e4  UpperLimitStiffnessUnits=N*m/deg  UpperLimitDamping=10  UpperLimitDampingUnits=N*m/(deg/s)  UpperLimitTransitionRegionWidth=0.1  UpperLimitTransitionRegionWidthUnits=deg  PositionTargetSpecify=on  PositionTargetPriority=High  PositionTargetValue=90  PositionTargetValueUnits=deg  VelocityTargetSpecify=off  VelocityTargetPriority=High  VelocityTargetValue=0  VelocityTargetValueUnits=deg/s
  Revolute Joint1 : sm_lib/Joints/Revolute Joint  Commented=on  JointMode=Normal  SenseConstraintForce=off  SenseConstraintForceX=off  SenseConstraintForceY=off  SenseConstraintForceZ=off  SenseConstraintTorque=off  SenseConstraintTorqueX=off  SenseConstraintTorqueY=off  SenseConstraintTorqueZ=off  SenseTotalForce=off  SenseTotalForceX=off  SenseTotalForceY=off  SenseTotalForceZ=off  SenseTotalTorque=off  SenseTotalTorqueX=off  SenseTotalTorqueY=off  SenseTotalTorqueZ=off  CompositeWrenchDir=FollowerOnBase  CompositeWrenchFrame=BaseFrame  EquilibriumPosition=0  EquilibriumPositionUnits=deg  SpringStiffness=0  SpringStiffnessUnits=N*m/deg  DampingCoefficient=0  DampingCoefficientUnits=N*m/(deg/s)  TorqueActuationMode=InputTorque  MotionActuationMode=ComputedMotion  SensePosition=off  SenseVelocity=on  SenseAcceleration=off  SenseTorqueForce=off  SenseLowerLimitTorqueForce=off  SenseUpperLimitTorqueForce=off  LowerLimitSpecify=off  LowerLimitBound=-90  LowerLimitBoundUnits=deg  LowerLimitStiffness=1e4  LowerLimitStiffnessUnits=N*m/deg  LowerLimitDamping=10  LowerLimitDampingUnits=N*m/(deg/s)  LowerLimitTransitionRegionWidth=0.1  LowerLimitTransitionRegionWidthUnits=deg  UpperLimitSpecify=off  UpperLimitBound=90  UpperLimitBoundUnits=deg  UpperLimitStiffness=1e4  UpperLimitStiffnessUnits=N*m/deg  UpperLimitDamping=10  UpperLimitDampingUnits=N*m/(deg/s)  UpperLimitTransitionRegionWidth=0.1  UpperLimitTransitionRegionWidthUnits=deg  PositionTargetSpecify=on  PositionTargetPriority=High  PositionTargetValue=90  PositionTargetValueUnits=deg  VelocityTargetSpecify=off  VelocityTargetPriority=High  VelocityTargetValue=0  VelocityTargetValueUnits=deg/s
  Revolute Joint4 : sm_lib/Joints/Revolute Joint  Commented=on  JointMode=Normal  SenseConstraintForce=off  SenseConstraintForceX=off  SenseConstraintForceY=off  SenseConstraintForceZ=off  SenseConstraintTorque=off  SenseConstraintTorqueX=off  SenseConstraintTorqueY=off  SenseConstraintTorqueZ=off  SenseTotalForce=off  SenseTotalForceX=off  SenseTotalForceY=off  SenseTotalForceZ=off  SenseTotalTorque=off  SenseTotalTorqueX=off  SenseTotalTorqueY=off  SenseTotalTorqueZ=off  CompositeWrenchDir=FollowerOnBase  CompositeWrenchFrame=BaseFrame  EquilibriumPosition=0  EquilibriumPositionUnits=deg  SpringStiffness=0  SpringStiffnessUnits=N*m/deg  DampingCoefficient=0  DampingCoefficientUnits=N*m/(deg/s)  TorqueActuationMode=InputTorque  MotionActuationMode=ComputedMotion  SensePosition=off  SenseVelocity=on  SenseAcceleration=off  SenseTorqueForce=off  SenseLowerLimitTorqueForce=off  SenseUpperLimitTorqueForce=off  LowerLimitSpecify=off  LowerLimitBound=-90  LowerLimitBoundUnits=deg  LowerLimitStiffness=1e4  LowerLimitStiffnessUnits=N*m/deg  LowerLimitDamping=10  LowerLimitDampingUnits=N*m/(deg/s)  LowerLimitTransitionRegionWidth=0.1  LowerLimitTransitionRegionWidthUnits=deg  UpperLimitSpecify=off  UpperLimitBound=90  UpperLimitBoundUnits=deg  UpperLimitStiffness=1e4  UpperLimitStiffnessUnits=N*m/deg  UpperLimitDamping=10  UpperLimitDampingUnits=N*m/(deg/s)  UpperLimitTransitionRegionWidth=0.1  UpperLimitTransitionRegionWidthUnits=deg  PositionTargetSpecify=on  PositionTargetPriority=High  PositionTargetValue=90  PositionTargetValueUnits=deg  VelocityTargetSpecify=off  VelocityTargetPriority=High  VelocityTargetValue=0  VelocityTargetValueUnits=deg/s
  Rigid Transform1 : sm_lib/Frames and Transforms/Rigid Transform  Commented=on  TranslationMethod=Cartesian  TranslationStandardOffset=45  TranslationLengthUnit=cm  TranslationStandardAxis=+Y  TranslationCartesianOffset=[0 1.7 0]  TranslationROffset=0  TranslationROffsetUnits=m  TranslationZOffset=0  TranslationZOffsetUnits=m  TranslationThetaOffset=0  TranslationThetaOffsetUnits=deg  RotationMethod=StandardAxis  RotationAngleUnits=deg  RotationStandardAxis=-X  RotationAngle=90  RotationArbitraryAxis=[0 0 1]  FollAlignAxisA=+X  BaseAlignAxisA=+Y  FollAlignAxisB=+Y  BaseAlignAxisB=+Z  RotationSequenceAxes=FollowerAxes  RotationSequence=XYX  RotationSequenceAngles=[0 0 0]  RotationSequenceAnglesUnits=deg  RotationMatrix=[1 0 0; 0 1 0; 0 0 1]  Quaternion=[1 0 0 0]
  Rigid Transform2 : sm_lib/Frames and Transforms/Rigid Transform  Commented=on  TranslationMethod=Cartesian  TranslationStandardOffset=45  TranslationLengthUnit=cm  TranslationStandardAxis=+Y  TranslationCartesianOffset=[0 0 -1.5]  TranslationROffset=0  TranslationROffsetUnits=m  TranslationZOffset=0  TranslationZOffsetUnits=m  TranslationThetaOffset=0  TranslationThetaOffsetUnits=deg  RotationMethod=StandardAxis  RotationAngleUnits=deg  RotationStandardAxis=+X  RotationAngle=90  RotationArbitraryAxis=[0 0 1]  FollAlignAxisA=+X  BaseAlignAxisA=+Y  FollAlignAxisB=+Y  BaseAlignAxisB=+Z  RotationSequenceAxes=FollowerAxes  RotationSequence=XYX  RotationSequenceAngles=[0 0 0]  RotationSequenceAnglesUnits=deg  RotationMatrix=[1 0 0; 0 1 0; 0 0 1]  Quaternion=[1 0 0 0]
  Rigid Transform3 : sm_lib/Frames and Transforms/Rigid Transform  Commented=on  TranslationMethod=Cartesian  TranslationStandardOffset=45  TranslationLengthUnit=cm  TranslationStandardAxis=+Y  TranslationCartesianOffset=[0 0 -10]  TranslationROffset=0  TranslationROffsetUnits=m  TranslationZOffset=0  TranslationZOffsetUnits=m  TranslationThetaOffset=0  TranslationThetaOffsetUnits=deg  RotationMethod=StandardAxis  RotationAngleUnits=deg  RotationStandardAxis=+Z  RotationAngle=90  RotationArbitraryAxis=[0 0 1]  FollAlignAxisA=+X  BaseAlignAxisA=+Y  FollAlignAxisB=+Y  BaseAlignAxisB=+Z  RotationSequenceAxes=FollowerAxes  RotationSequence=XYX  RotationSequenceAngles=[0 0 0]  RotationSequenceAnglesUnits=deg  RotationMatrix=[1 0 0; 0 1 0; 0 0 1]  Quaternion=[1 0 0 0]
  Rigid Transform4 : sm_lib/Frames and Transforms/Rigid Transform  Commented=on  TranslationMethod=Cartesian  TranslationStandardOffset=45  TranslationLengthUnit=cm  TranslationStandardAxis=+Y  TranslationCartesianOffset=[0 0 -1]  TranslationROffset=0  TranslationROffsetUnits=m  TranslationZOffset=0  TranslationZOffsetUnits=m  TranslationThetaOffset=0  TranslationThetaOffsetUnits=deg  RotationMethod=StandardAxis  RotationAngleUnits=deg  RotationStandardAxis=+X  RotationAngle=90  RotationArbitraryAxis=[0 0 1]  FollAlignAxisA=+X  BaseAlignAxisA=+Y  FollAlignAxisB=+Y  BaseAlignAxisB=+Z  RotationSequenceAxes=FollowerAxes  RotationSequence=XYX  RotationSequenceAngles=[0 0 0]  RotationSequenceAnglesUnits=deg  RotationMatrix=[1 0 0; 0 1 0; 0 0 1]  Quaternion=[1 0 0 0]
  Rigid Transform5 : sm_lib/Frames and Transforms/Rigid Transform  Commented=on  TranslationMethod=Cartesian  TranslationStandardOffset=90  TranslationLengthUnit=cm  TranslationStandardAxis=-Y  TranslationCartesianOffset=[0 1.5 0]  TranslationROffset=0  TranslationROffsetUnits=m  TranslationZOffset=0  TranslationZOffsetUnits=m  TranslationThetaOffset=90  TranslationThetaOffsetUnits=deg  RotationMethod=StandardAxis  RotationAngleUnits=deg  RotationStandardAxis=-X  RotationAngle=90  RotationArbitraryAxis=[0 0 1]  FollAlignAxisA=+X  BaseAlignAxisA=+Y  FollAlignAxisB=+Y  BaseAlignAxisB=+Z  RotationSequenceAxes=FollowerAxes  RotationSequence=XYX  RotationSequenceAngles=[0 0 0]  RotationSequenceAnglesUnits=deg  RotationMatrix=[1 0 0; 0 1 0; 0 0 1]  Quaternion=[1 0 0 0]
  Saturation1 : Saturate  UpperLimit=11.5  LowerLimit=-11.5
  Saturation10 : Saturate  UpperLimit=11.5  LowerLimit=-11.5
  Saturation{2..5} (4 alike) : Saturate  UpperLimit=11.5  LowerLimit=0
  Saturation6 : Saturate  Commented=on  UpperLimit=11.5  LowerLimit=-11.5
  Saturation7 : Saturate  Commented=on  UpperLimit=11.5  LowerLimit=-11.5
  Saturation8 : Saturate  UpperLimit=11.5  LowerLimit=-11.5
  Saturation9 : Saturate  Commented=on  UpperLimit=11.5  LowerLimit=-11.5
  Scope{,1..3,6,10..16} (12 alike) : Scope
  Scope5 : Scope  Commented=on
  Simulink-PS Converter{,1..3} (4 alike) : nesl_utility/Simulink-PS Converter  Commented=on  PhysicalDomain=network_engine_domain  SubClassName=ps_input  LeftPortType=input  RightPortType=output  PseudoPeriodic=off  Frequencies=[]  NoiseDistribution=none  NoiseParameters=[]  Unit=1  AffineConversion=off  FilteringAndDerivatives=zero  SimscapeFilterOrder=1  InputFilterTimeConstant=0.001  UdotUserProvided=1
  Simulink-PS Converter10 : nesl_utility/Simulink-PS Converter  Commented=on  PhysicalDomain=network_engine_domain  SubClassName=ps_input  LeftPortType=input  RightPortType=output  PseudoPeriodic=off  Frequencies=[]  NoiseDistribution=none  NoiseParameters=[]  Unit=1  AffineConversion=off  FilteringAndDerivatives=provide  SimscapeFilterOrder=1  InputFilterTimeConstant=0.001  UdotUserProvided=0
  Simulink-PS Converter{4..9} (6 alike) : nesl_utility/Simulink-PS Converter  Commented=on  PhysicalDomain=network_engine_domain  SubClassName=ps_input  LeftPortType=input  RightPortType=output  PseudoPeriodic=off  Frequencies=[]  NoiseDistribution=none  NoiseParameters=[]  Unit=1  AffineConversion=off  FilteringAndDerivatives=filter  SimscapeFilterOrder=2  InputFilterTimeConstant=0.002  UdotUserProvided=0
  Slider Gain : simulink/Math Operations/Slider Gain  Commented=on  gain=0  low=0  high=500
  Solver Configuration : nesl_utility/Solver Configuration  Commented=on  PhysicalDomain=network_engine_domain  SubClassName=solver  LeftPortType=input  RightPortType=generic  Tones=[]  Harmonics=[]  SimulateNoise=off  Profile=off  UseLocalSampling=off  EnableSwitchedLinearOptims=on  FrequencyDomain=off  UseCCode=off  RelTol=0.001  AbsTol=1e-06  MinStep=1e-09  ToWorkspace=off  RevertToSquareIcSolve=off  NumHomotopyIterations=100  PhasorMode=off  PhasorModeNumHarmonics=1  ConsistencySolver=NEWTON_FTOL  IndexReductionMethod=DerivativeReplacement  DoDC=off  ResidualTolerance=1e-09  ConsistencyTolSource=GLOBAL  ConsistencyAbsTol=0.001  ConsistencyRelTol=0.001  ConsistencyTolFactor=0.001  UseLocalSolver=off  LocalSolverChoice=NE_BACKWARD_EULER_ADVANCER  ResolveIndetEquations=on  FunctionEvalNumThread=1  LocalSolverSampleTime=0.001  DoFixedCost=off  MaxNonlinIter=3  MaxModeIter=2  ComputeImpulses=off  ImpulseIterations=2  LinearAlgebra=Sparse  LinearAlgebraNumThread=0  EquationFormulation=NE_TIME_EF  DelaysMemoryBudget=1024  AutomaticFiltering=on  FilteringTimeConstant=0.001  PartitionStorageMethod=AS_NEEDED  PartitionMemoryBudget=1024  PartitionMethod=FAST
  State : Scope  NumInputPorts=2
  Subsystem4 : Subsystem
  Sum : Sum  Inputs=|++
  Sum{1..4,9..10,12,19..20} (9 alike) : Sum  Inputs=|+-
  Sum11 : Sum  Inputs=|++
  Sum{7..8,13..18} (8 alike) : Sum  Commented=on  Inputs=|+-
  Transform Arm Ref : sm_lib/Frames and Transforms/Rigid Transform  Commented=on  TranslationMethod=Cartesian  TranslationStandardOffset=0  TranslationLengthUnit=mm  TranslationStandardAxis=+Z  TranslationCartesianOffset=[0 0 -26]  TranslationROffset=0  TranslationROffsetUnits=m  TranslationZOffset=0  TranslationZOffsetUnits=m  TranslationThetaOffset=0  TranslationThetaOffsetUnits=deg  RotationMethod=StandardAxis  RotationAngleUnits=deg  RotationStandardAxis=+Z  RotationAngle=90  RotationArbitraryAxis=[0 0 1]  FollAlignAxisA=+X  BaseAlignAxisA=+Y  FollAlignAxisB=+Y  BaseAlignAxisB=+Z  RotationSequenceAxes=FollowerAxes  RotationSequence=XYX  RotationSequenceAngles=[0 0 0]  RotationSequenceAnglesUnits=deg  RotationMatrix=[1 0 0; 0 1 0; 0 0 1]  Quaternion=[1 0 0 0]
  Transform Arm1 : sm_lib/Frames and Transforms/Rigid Transform  Commented=on  TranslationMethod=Cartesian  TranslationStandardOffset=0  TranslationLengthUnit=mm  TranslationStandardAxis=+Z  TranslationCartesianOffset=[12 58 -38]  TranslationROffset=0  TranslationROffsetUnits=m  TranslationZOffset=0  TranslationZOffsetUnits=m  TranslationThetaOffset=0  TranslationThetaOffsetUnits=deg  RotationMethod=RotationSequence  RotationAngleUnits=deg  RotationStandardAxis=+Z  RotationAngle=0  RotationArbitraryAxis=[0 0 1]  FollAlignAxisA=+X  BaseAlignAxisA=+Y  FollAlignAxisB=+Y  BaseAlignAxisB=+Z  RotationSequenceAxes=FollowerAxes  RotationSequence=ZXZ  RotationSequenceAngles=[0 90 0]  RotationSequenceAnglesUnits=deg  RotationMatrix=[1 0 0; 0 1 0; 0 0 1]  Quaternion=[1 0 0 0]
  Transform Arm2 : sm_lib/Frames and Transforms/Rigid Transform  Commented=on  TranslationMethod=Cartesian  TranslationStandardOffset=0  TranslationLengthUnit=mm  TranslationStandardAxis=+Z  TranslationCartesianOffset=[58 -12 -38]  TranslationROffset=0  TranslationROffsetUnits=m  TranslationZOffset=0  TranslationZOffsetUnits=m  TranslationThetaOffset=0  TranslationThetaOffsetUnits=deg  RotationMethod=RotationSequence  RotationAngleUnits=deg  RotationStandardAxis=+Z  RotationAngle=-90  RotationArbitraryAxis=[0 0 1]  FollAlignAxisA=+X  BaseAlignAxisA=+Y  FollAlignAxisB=+Y  BaseAlignAxisB=+Z  RotationSequenceAxes=FollowerAxes  RotationSequence=ZXZ  RotationSequenceAngles=[-90 90 0]  RotationSequenceAnglesUnits=deg  RotationMatrix=[1 0 0; 0 1 0; 0 0 1]  Quaternion=[1 0 0 0]
  Transform Arm3 : sm_lib/Frames and Transforms/Rigid Transform  Commented=on  TranslationMethod=Cartesian  TranslationStandardOffset=0  TranslationLengthUnit=mm  TranslationStandardAxis=+Z  TranslationCartesianOffset=[-58 12 -38]  TranslationROffset=0  TranslationROffsetUnits=m  TranslationZOffset=0  TranslationZOffsetUnits=m  TranslationThetaOffset=0  TranslationThetaOffsetUnits=deg  RotationMethod=RotationSequence  RotationAngleUnits=deg  RotationStandardAxis=+Z  RotationAngle=90  RotationArbitraryAxis=[0 0 1]  FollAlignAxisA=+X  BaseAlignAxisA=+Y  FollAlignAxisB=+Y  BaseAlignAxisB=+Z  RotationSequenceAxes=FollowerAxes  RotationSequence=ZXZ  RotationSequenceAngles=[90 90 0]  RotationSequenceAnglesUnits=deg  RotationMatrix=[1 0 0; 0 1 0; 0 0 1]  Quaternion=[1 0 0 0]
  Transform Arm4 : sm_lib/Frames and Transforms/Rigid Transform  Commented=on  TranslationMethod=Cartesian  TranslationStandardOffset=0  TranslationLengthUnit=mm  TranslationStandardAxis=+Z  TranslationCartesianOffset=[-12 -58 -38]  TranslationROffset=0  TranslationROffsetUnits=m  TranslationZOffset=0  TranslationZOffsetUnits=m  TranslationThetaOffset=0  TranslationThetaOffsetUnits=deg  RotationMethod=RotationSequence  RotationAngleUnits=deg  RotationStandardAxis=+Z  RotationAngle=180  RotationArbitraryAxis=[0 0 1]  FollAlignAxisA=+X  BaseAlignAxisA=+Y  FollAlignAxisB=+Y  BaseAlignAxisB=+Z  RotationSequenceAxes=FollowerAxes  RotationSequence=ZXZ  RotationSequenceAngles=[180 90 0]  RotationSequenceAnglesUnits=deg  RotationMatrix=[1 0 0; 0 1 0; 0 0 1]  Quaternion=[1 0 0 0]
  Transform Leg Right : sm_lib/Frames and Transforms/Rigid Transform  Commented=on  TranslationMethod=Cartesian  TranslationStandardOffset=0.09-drone_leg.width/2  TranslationLengthUnit=m  TranslationStandardAxis=-Y  TranslationCartesianOffset=[0 -0.08 -0.001]  TranslationROffset=0  TranslationROffsetUnits=m  TranslationZOffset=0  TranslationZOffsetUnits=m  TranslationThetaOffset=0  TranslationThetaOffsetUnits=deg  RotationMethod=StandardAxis  RotationAngleUnits=deg  RotationStandardAxis=-X  RotationAngle=180  RotationArbitraryAxis=[0 0 1]  FollAlignAxisA=+X  BaseAlignAxisA=+Y  FollAlignAxisB=+Y  BaseAlignAxisB=+Z  RotationSequenceAxes=FollowerAxes  RotationSequence=XYX  RotationSequenceAngles=[0 0 0]  RotationSequenceAnglesUnits=deg  RotationMatrix=[1 0 0; 0 1 0; 0 0 1]  Quaternion=[1 0 0 0]
  Transform Leg Right1 : sm_lib/Frames and Transforms/Rigid Transform  Commented=on  TranslationMethod=Cartesian  TranslationStandardOffset=0.09-drone_leg.width/2  TranslationLengthUnit=m  TranslationStandardAxis=-Y  TranslationCartesianOffset=[0 0.08 -0.001]  TranslationROffset=0  TranslationROffsetUnits=m  TranslationZOffset=0  TranslationZOffsetUnits=m  TranslationThetaOffset=0  TranslationThetaOffsetUnits=deg  RotationMethod=StandardAxis  RotationAngleUnits=deg  RotationStandardAxis=-X  RotationAngle=180  RotationArbitraryAxis=[0 0 1]  FollAlignAxisA=+X  BaseAlignAxisA=+Y  FollAlignAxisB=+Y  BaseAlignAxisB=+Z  RotationSequenceAxes=FollowerAxes  RotationSequence=XYX  RotationSequenceAngles=[0 0 0]  RotationSequenceAnglesUnits=deg  RotationMatrix=[1 0 0; 0 1 0; 0 0 1]  Quaternion=[1 0 0 0]
  Transform Propeller{1..4} (4 alike) : sm_lib/Frames and Transforms/Rigid Transform  Commented=on  TranslationMethod=Cartesian  TranslationStandardOffset=0  TranslationLengthUnit=mm  TranslationStandardAxis=+Z  TranslationCartesianOffset=[0 0 -20]  TranslationROffset=0  TranslationROffsetUnits=m  TranslationZOffset=0  TranslationZOffsetUnits=m  TranslationThetaOffset=0  TranslationThetaOffsetUnits=deg  RotationMethod=StandardAxis  RotationAngleUnits=deg  RotationStandardAxis=-X  RotationAngle=90  RotationArbitraryAxis=[0 0 1]  FollAlignAxisA=+X  BaseAlignAxisA=+Y  FollAlignAxisB=+Y  BaseAlignAxisB=+Z  RotationSequenceAxes=FollowerAxes  RotationSequence=XYX  RotationSequenceAngles=[0 0 0]  RotationSequenceAnglesUnits=deg  RotationMatrix=[1 0 0; 0 1 0; 0 0 1]  Quaternion=[1 0 0 0]
  Transform{1..4} (4 alike) : sm_lib/Frames and Transforms/Rigid Transform  Commented=on  TranslationMethod=StandardAxis  TranslationStandardOffset=0.0097  TranslationLengthUnit=m  TranslationStandardAxis=+Y  TranslationCartesianOffset=[0 0 5]  TranslationROffset=0  TranslationROffsetUnits=m  TranslationZOffset=0  TranslationZOffsetUnits=m  TranslationThetaOffset=0  TranslationThetaOffsetUnits=deg  RotationMethod=None  RotationAngleUnits=deg  RotationStandardAxis=+X  RotationAngle=-90  RotationArbitraryAxis=[0 0 1]  FollAlignAxisA=+X  BaseAlignAxisA=+Y  FollAlignAxisB=+Y  BaseAlignAxisB=+Z  RotationSequenceAxes=FollowerAxes  RotationSequence=XYX  RotationSequenceAngles=[0 0 0]  RotationSequenceAnglesUnits=deg  RotationMatrix=[1 0 0; 0 1 0; 0 0 1]  Quaternion=[1 0 0 0]
  World : sm_lib/Frames and Transforms/World Frame  Commented=on
  base : sm_lib/Body Elements/Brick Solid  Commented=on  GraphicAmbientColor=[0.15 0.9 0.15 1.0]  BasedOnType=Density  BrickDimensions=[100 100 1]  BrickDimensionUnits=cm  CenterOfMass=[0 0 0]  CenterOfMassUnits=m  GraphicDiffuseColor=[0.0 0.8 0.0]  Density=1000  DensityUnits=kg/(m^3)  DoExposeReferenceFrame=on  GraphicEmissiveColor=[0.0 0.0 0.0 1.0]  ExportEntireGeometry=off  SerializedFrames=<Frames/>  MarkerShape=Sphere  MarkerSize=10  GraphicType=FromGeometry  InertiaType=CalculateFromGeometry  Mass=1  MassUnits=kg  MomentsOfInertia=[1 1 1]  MomentsOfInertiaUnits=kg*m^2  GraphicOpacity=1.0  ProductsOfInertia=[0 0 0]  ProductsOfInertiaUnits=kg*m^2  GraphicShininess=75  GraphicSpecularColor=[0.5 0.5 0.5 1.0]  GraphicVisPropType=SimpleVisualProperties
  plate_top 1 : sm_lib/Body Elements/File Solid  Commented=on  ExtGeomFileName=C:\Users\tridu\OneDrive\Máy tính\Code Matlad\quadcopter\CAD\Geometry\Part3.STEP  UnitType=FromFile  ExtGeomFileUnits=m  StepReaderType=HEX  ExportConvexHullGeometry=off  InertiaType=Custom  Mass=0.0317292  MassUnits=kg  CenterOfMass=[9.57262e-08, 1.0716e-07, -1.47882e-10]  CenterOfMassUnits=m  MomentsOfInertia=[2.77785e-05, 2.75764e-05, 5.53432e-05]  MomentsOfInertiaUnits=kg*m^2  ProductsOfInertia=[-9.24719e-13, -9.71809e-13, 1.0181e-10]  ProductsOfInertiaUnits=kg*m^2  BasedOnType=Density  Density=1  DensityUnits=g/cm^3  DoExposeReferenceFrame=on  SerializedFrames=<Frames/>  GraphicType=FromGeometry  MarkerShape=Sphere  MarkerSize=10  GraphicVisPropType=FromFileVisualProperties  GraphicDiffuseColor=[0.0 0.0 0.0]  GraphicSpecularColor=[0.5 0.5 0.5 1.0]  GraphicAmbientColor=[0.15 0.15 0.15 1.0]  GraphicEmissiveColor=[0.0 0.0 0.0 1.0]  GraphicShininess=75  GraphicOpacity=1.0
  plate_top 2 : sm_lib/Body Elements/File Solid  Commented=on  ExtGeomFileName=C:\Users\tridu\OneDrive\Máy tính\Code Matlad\quadcopter\CAD\Geometry\Part3.STEP  UnitType=FromFile  ExtGeomFileUnits=m  StepReaderType=HEX  ExportConvexHullGeometry=off  InertiaType=Custom  Mass=0.0317292  MassUnits=kg  CenterOfMass=[9.57262e-08, 1.0716e-07, -1.47882e-10]  CenterOfMassUnits=m  MomentsOfInertia=[2.77785e-05, 2.75764e-05, 5.53432e-05]  MomentsOfInertiaUnits=kg*m^2  ProductsOfInertia=[-9.24719e-13, -9.71809e-13, 1.0181e-10]  ProductsOfInertiaUnits=kg*m^2  BasedOnType=Density  Density=1  DensityUnits=g/cm^3  DoExposeReferenceFrame=on  SerializedFrames=<Frames/>  GraphicType=FromGeometry  MarkerShape=Sphere  MarkerSize=10  GraphicVisPropType=FromFileVisualProperties  GraphicDiffuseColor=[0.0 0.0 0.0]  GraphicSpecularColor=[0.5 0.5 0.5 1.0]  GraphicAmbientColor=[0.15 0.15 0.15 1.0]  GraphicEmissiveColor=[0.0 0.0 0.0 1.0]  GraphicShininess=75  GraphicOpacity=1.0
  tag scope: D1=global, D2=global, D3=global, D4=global, HS_MSKK=global, T1=global, T2=global, T3=global, T4=global, U1=global, U2=global, U3=global, U4=global, pitch=global, pitchdot=global, roll=global, rolldot=global, x2dot=global, x=global, x_SP=global, xdot=global, y2dot=global, y=global, y_SP=global, yaw=global, yawdot=global, ydot=global, z=global, z_SP=global, zdot=global
  wires:
  Integrator8/1 -> [pitchdot], Integrator9/1
  From19/1 -> Simulink-PS Converter5/1
  [roll] -> MATLAB Function/5(roll)
  [ydot] -> MATLAB Function/13(y_dot)
  [T2] -> MATLAB Function/2(T2)
  Integrator11/1 -> [yaw]
  Gain6/1 -> Mux2/3
  Constant37/1 -> Simulink-PS Converter2/1
  [pitchdot] -> Mux3/2
  HS_MSKK/1 -> [HS_MSKK]
  [yaw] -> Gain6/1
  [z] -> Mux/3
  Add4/1 -> Saturation4/1
  Mux2/1 -> State/2, Scope2/1
  [yaw] -> MATLAB Function/7(yaw)
  Constant38/1 -> Simulink-PS Converter3/1
  Add5/1 -> Saturation5/1
  [zdot] -> MATLAB Function/14(z_dot)
  [ydot] -> Mux1/2
  [pitch] -> MATLAB Function/6(pitch)
  [y] -> Mux/2
  Constant/1 -> Add4/1, Add5/1, Add3/1, Add1/1
  [rolldot] -> Mux3/1
  Integrator6/1 -> [rolldot], Integrator7/1
  [T3] -> MATLAB Function/3(T3)
  Gain4/1 -> Mux2/1
  [roll] -> Gain4/1
  [rolldot] -> MATLAB Function/8(roll_dot)
  Gain5/1 -> Mux2/2
  Integrator1/1 -> [x]
  [pitchdot] -> MATLAB Function/9(pitch_dot)
  [xdot] -> Mux1/1
  Mux3/1 -> Scope3/1
  Integrator7/1 -> [roll]
  Mux1/1 -> Scope1/1
  Integrator3/1 -> [y]
  Integrator4/1 -> [zdot], Integrator5/1
  [zdot] -> Mux1/3
  Integrator10/1 -> [yawdot], Integrator11/1
  Integrator/1 -> [xdot], Integrator1/1
  MATLAB Function/3(z2dot) -> Integrator4/1
  [x] -> Mux/1
  MATLAB Function/2(y2dot) -> [y2dot], Integrator2/1
  [T4] -> MATLAB Function/4(T4)
  [pitch] -> Gain5/1
  [yawdot] -> Mux3/3
  MATLAB Function/4(roll2dot) -> Integrator6/1
  [HS_MSKK] -> MATLAB Function/11(HS_MSKK)
  Mux/1 -> State/1, Scope/1
  From20/1 -> Simulink-PS Converter6/1
  [yawdot] -> MATLAB Function/10(yaw_dot)
  Integrator9/1 -> [pitch]
  Add1/1 -> Saturation2/1
  From21/1 -> Simulink-PS Converter7/1
  MATLAB Function/5(pitch2dot) -> Integrator8/1
  Integrator2/1 -> [ydot], Integrator3/1
  [xdot] -> MATLAB Function/12(x_dot)
  Add3/1 -> Saturation3/1
  Integrator5/1 -> [z]
  [U1] -> Gain8/1
  [U1] -> Gain9/1
  [U1] -> Gain10/1
  [U1] -> Gain12/1
  [U2] -> Gain13/1
  [U2] -> Gain19/1
  [U4] -> Gain18/1
  [U3] -> Gain17/1
  [U4] -> Gain16/1
  [U4] -> Gain11/1
  [U4] -> Gain14/1
  [U3] -> Gain15/1
  Gain8/1 -> Add1/2
  Gain9/1 -> Add3/2
  Gain10/1 -> Add4/2
  Gain12/1 -> Add5/2
  Gain11/1 -> Add3/3
  Gain13/1 -> Add3/4
  Gain14/1 -> Add1/3
  Gain15/1 -> Add1/4
  Gain16/1 -> Add4/3
  Gain17/1 -> Add4/4
  Gain18/1 -> Add5/3
  Gain19/1 -> Add5/4
  Constant4/1 -> Sum7/1
  Constant16/1 -> Sum15/1
  Constant17/1 -> Sum16/1
  Constant15/1 -> Sum14/1
  From60/1 -> Sum8/2
  From57/1 -> Sum7/2
  From22/1 -> Sum13/2
  From29/1 -> Sum18/2
  From28/1 -> Sum17/2
  From27/1 -> Sum14/2
  From26/1 -> Sum15/2
  From23/1 -> Sum16/2
  Mux5/1 -> Gain21/1
  Sum8/1 -> Mux5/1
  Sum7/1 -> Mux5/2
  Sum13/1 -> Mux5/3
  Sum14/1 -> Mux5/6
  Sum15/1 -> Mux5/7
  Sum16/1 -> Mux5/8
  Saturation6/1 -> Gain22/1
  Saturation7/1 -> Gain23/1
  Gain22/1 -> Goto22/1
  Gain23/1 -> Goto23/1
  Gain3/1 -> Simulink-PS Converter4/1
  From25/1 -> Gain2/1
  From24/1 -> Gain3/1
  Gain2/1 -> Simulink-PS Converter9/1
  MATLAB Function1/2(T2) -> Mux4/2, [T2]
  MATLAB Function1/3(T3) -> Mux4/3, [T3]
  MATLAB Function1/4(T4) -> Mux4/4, [T4]
  [D4] -> MATLAB Function1/4(D4)
  [D3] -> MATLAB Function1/3(D3)
  [D2] -> MATLAB Function1/2(D2)
  [D1] -> MATLAB Function1/1(D1)
  Saturation5/1 -> MATLAB Function2/4(T4)
  Saturation2/1 -> MATLAB Function2/1(T1)
  Saturation3/1 -> MATLAB Function2/2(T2)
  Saturation4/1 -> MATLAB Function2/3(T3)
  MATLAB Function2/1(D1) -> Display/1, [D1]
  MATLAB Function2/3(D3) -> Display2/1, [D3]
  MATLAB Function2/4(D4) -> Display3/1, [D4]
  MATLAB Function2/2(D2) -> Display1/1, [D2]
  MATLAB Function1/1(T1) -> Mux4/1, [T1]
  Demux1/1 -> Giới hạn công suất U1/1
  Saturation9/1 -> Gain25/1
  Gain25/1 -> Goto29/1
  Demux1/4 -> Saturation9/1
  Demux1/3 -> Saturation7/1
  Sum17/1 -> Mux5/5
  Sum18/1 -> Mux5/4
  Constant14/1 -> Sum17/1
  Constant13/1 -> Sum8/1
  Gain21/1 -> Scope5/1, Demux1/1
  Constant1/1 -> Simulink-PS Converter/1
  Constant7/1 -> Simulink-PS Converter1/1
  Giới hạn công suất U1/1 -> Goto21/1
  Mux4/1 -> Scope6/1
  Demux1/2 -> Saturation6/1
  MATLAB Function/1(x2dot) -> [x2dot], Integrator/1
  MATLAB Function/6(yaw2dot) -> Integrator10/1
  From72/1 -> Sum18/1
  From71/1 -> Sum13/1
  Demux2/2 -> Saturation1/1
  Giới hạn công suất U2/1 -> [U1]
  Gain7/1 -> Demux2/1, Scope10/1
  Constant3/1 -> Sum9/1
  Demux2/3 -> Saturation8/1
  Demux2/4 -> Saturation10/1
  Gain26/1 -> [U4]
  Saturation10/1 -> Gain26/1
  Gain24/1 -> [U3]
  Gain20/1 -> [U2]
  Saturation8/1 -> Gain24/1
  Saturation1/1 -> Gain20/1
  Mux10/1 -> Gain7/1
  [yawdot] -> Sum4/2
  [pitchdot] -> Sum3/2
  [rolldot] -> Sum2/2
  [yaw] -> Sum9/2
  [pitch] -> Sum10/2
  [roll] -> Sum1/2
  Constant23/1 -> Sum2/1
  Constant26/1 -> Sum4/1
  Constant25/1 -> Sum3/1
  Sum1/1 -> Mux10/1
  Sum10/1 -> Mux10/2
  Sum9/1 -> Mux10/3
  Sum2/1 -> Mux10/4
  Sum3/1 -> Mux10/5
  Sum4/1 -> Mux10/6
  From18/1 -> Gain1/1
  Gain1/1 -> Simulink-PS Converter8/1
  Constant28/1 -> Slider Gain/1
  Slider Gain/1 -> Gain27/1
  Gain27/1 -> Simulink-PS Converter10/1
  Demux2/1 -> Add/2
  Add/1 -> Giới hạn công suất U2/1
  [U1] -> Mux11/1
  [U2] -> Mux11/2
  [U3] -> Mux11/3
  [U4] -> Mux11/4
  Mux11/1 -> Scope11/1
  [U1] -> Display4/1
  [U2] -> Display5/1
  [U3] -> Display6/1
  [U4] -> Display7/1
  [Uz] -> Add/1
  [T1] -> MATLAB Function/1(T1)
  [T1] -> Display14/1
  [T4] -> Display17/1
  [T2] -> Display15/1
  [T3] -> Display16/1
  [x] -> Display8/1
  [y] -> Display9/1
  [z] -> Display10/1
  Mux12/1 -> Scope12/1
  Constant27/1 -> Sum/1
  Sum/1 -> Sum1/1
  Constant2/1 -> Sum11/1
  Sum11/1 -> Sum10/1
  [pitch_SP] -> Sum11/2
  [roll_SP] -> Sum/2
  [Ux] -> Mux13/1
  [Uy] -> Mux13/2
  Mux13/1 -> Scope13/1
  [Uz] -> Mux13/3
  Mux14/1 -> Scope14/1
  [z] -> Mux14/3
  [x] -> Mux14/1
  [y] -> Mux14/2
  Mux15/1 -> Scope15/1
  [pitch] -> Gain29/1
  [yaw] -> Gain30/1
  Gain29/1 -> Mux15/2
  Gain30/1 -> Mux15/3
  Gain28/1 -> Mux15/1
  [roll] -> Gain28/1
  Constant36/1 -> [x_SP]
  Constant29/1 -> [y_SP]
  Constant31/1 -> [z_SP]
  [x] -> Sum12/2
  [y] -> Sum19/2
  [z] -> Sum20/2
  Sum20/1 -> Mux16/3
  Sum19/1 -> Mux16/2
  Sum12/1 -> Mux16/1
  Mux16/1 -> Scope16/1
  [z_SP] -> Sum20/1
  [y_SP] -> Sum19/1
  [x_SP] -> Sum12/1
  Subsystem4/1(Roll SP) -> Mux12/1
  Subsystem4/2(Pitch SP) -> Mux12/2
  connections:
  Transform Arm2/LConn1 -- Transform Arm4/LConn1 -- Transform Arm Ref/LConn1 -- Transform Arm1/LConn1 -- Transform Arm3/LConn1
  base/RConn1 -- MechanismConfiguration/RConn1 -- Solver Configuration/RConn1 -- Rigid Transform3/RConn1 -- World/RConn1
  Bushing Joint/RConn1 -- Transform Leg Right/LConn1 -- Transform Leg Right1/LConn1 -- Body/LConn1
  Arm2/RConn1 -- Rigid Transform5/LConn1
  Housing3/LConn1 -- Revolute Joint/RConn1
  Bushing Joint/LConn5 -- Simulink-PS Converter5/RConn1
  Transform1/LConn1 -- Propeller1/LConn1
  Transform Propeller2/LConn1 -- Housing2/RConn1
  Cap3/RConn1 -- Transform3/RConn1
  Propeller3/RConn1 -- Transform Propeller4/RConn1
  Cap2/RConn1 -- Transform2/RConn1
  Propeller4/RConn1 -- Transform Propeller3/RConn1
  Bushing Joint/LConn7 -- Simulink-PS Converter7/RConn1
  " Arm1"/RConn1 -- Rigid Transform2/RConn1
  Transform Arm3/RConn1 -- " Arm2"/LConn1
  Transform Propeller1/LConn1 -- Housing1/RConn1
  Rigid Transform1/RConn1 -- Revolute Joint/LConn1
  Rigid Transform2/LConn1 -- Revolute Joint1/LConn1
  plate_top 2/RConn1 -- Transform Leg Right1/RConn1
  Transform Propeller3/LConn1 -- Housing3/RConn1
  Rigid Transform4/LConn1 -- Revolute Joint4/LConn1
  Transform Propeller4/LConn1 -- Housing4/RConn1
  Bushing Joint/LConn6 -- Simulink-PS Converter6/RConn1
  Bushing Joint/LConn1 -- Rigid Transform3/LConn1
  Revolute Joint/LConn2 -- Simulink-PS Converter/RConn1
  Housing4/LConn1 -- Revolute Joint1/RConn1
  Cap1/RConn1 -- Transform1/RConn1
  Rigid Transform4/RConn1 -- " Arm2"/RConn1
  Transform Arm1/RConn1 -- Arm2/LConn1
  Arm1/RConn1 -- Rigid Transform1/LConn1
  Body/RConn1 -- Transform Arm Ref/RConn1
  Transform3/LConn1 -- Propeller4/LConn1
  Housing2/LConn1 -- Revolute Joint4/RConn1
  Revolute Joint3/LConn1 -- Rigid Transform5/RConn1
  Simulink-PS Converter2/RConn1 -- Revolute Joint3/LConn2
  Arm1/LConn1 -- Transform Arm4/RConn1
  Simulink-PS Converter1/RConn1 -- Revolute Joint1/LConn2
  Propeller1/RConn1 -- Transform Propeller1/RConn1
  Propeller2/RConn1 -- Transform Propeller2/RConn1
  plate_top 1/RConn1 -- Transform Leg Right/RConn1
  Transform4/LConn1 -- Propeller3/LConn1
  Transform2/LConn1 -- Propeller2/LConn1
  Housing1/LConn1 -- Revolute Joint3/RConn1
  Cap4/RConn1 -- Transform4/RConn1
  Revolute Joint4/LConn2 -- Simulink-PS Converter3/RConn1
  Transform Arm2/RConn1 -- " Arm1"/LConn1
  Bushing Joint/LConn4 -- Simulink-PS Converter8/RConn1
  Bushing Joint/LConn3 -- Simulink-PS Converter9/RConn1
  Bushing Joint/LConn2 -- Simulink-PS Converter4/RConn1
